simulink model "SteeringWheel"  (R2024b)
settings: configuration reference "STM32H7_Config" (kept outside this file)
libraries: simulink x3
(part 2 of 2)

== stateflow chart SteeringWheel/Overwrite System/BEMSOn ==
  state Map12
    entry:
    BEMSOnOW = 1;
  state Map11
    entry, during:
    BEMSOnOW = 0;
  state Map13
    entry, during:
    BEMSOnOW = -1;
  Map13 -> Map12 [order 2] : after(500,tick)
      | [BSteeringWheelButton3 ==1]
  Map11 -> Map12 [order 1] : after(500,tick)
      | [BSteeringWheelButton4 == 1]
  (default) -> Map13
  Map13 -> Map11 [order 1] : after(500,tick)
      | [BSteeringWheelButton4 ==1]
  Map12 -> Map13 [order 2] : after(500,tick)
      | [BSteeringWheelButton4 ==1]
  Map12 -> Map11 [order 1] : after(500,tick)
      | [BSteeringWheelButton3 == 1]
  Map11 -> Map13 [order 2] : after(500,tick)
      | [BSteeringWheelButton3 ==1]
  data: BSteeringWheelButton3 input double; BSteeringWheelButton4 input double; BEMSOnOW output double

== stateflow chart SteeringWheel/Overwrite System/NThrottleMap ==
  state Map14
    entry:
    NThrottleMapOW = -1;
    PDischargeMaxOW = -1;
    rTorqueSplitOW = -1;
  state Map12
    entry:
    NThrottleMapOW = 1;
    PDischargeMaxOW = 5;
    rTorqueSplitOW = 0.5;
  state Map7
    entry, during:
    NThrottleMapOW = 2;
    PDischargeMaxOW = 78;
    rTorqueSplitOW = 0.8;
  state Map8
    entry, during:
    NThrottleMapOW = 3;
    PDischargeMaxOW = 78;
    rTorqueSplitOW = 0.7;
  state Map9
    entry, during:
    NThrottleMapOW = 4;
    PDischargeMaxOW = 58;
    rTorqueSplitOW = 1;
  state Map10
    entry, during:
    NThrottleMapOW = 5;
    PDischargeMaxOW = 58;
    rTorqueSplitOW = 0.7;
  state Map13
    entry, during:
    NThrottleMapOW = 6;
    PDischargeMaxOW = 38;
    rTorqueSplitOW = 0.7;
  Map8 -> Map9 [order 2] : after(500,tick)
      | [BSteeringWheelButton3 == 1]
  Map10 -> Map13 [order 2] : after(500,tick)
      | [BSteeringWheelButton3 == 1]
  Map9 -> Map10 [order 2] : after(500,tick)
      | [BSteeringWheelButton3 == 1]
  Map7 -> Map8 [order 2] : after(500,tick)
      | [BSteeringWheelButton3 == 1]
  (default) -> Map14
  Map12 -> Map7 [order 2] : after(500,tick)
      | [BSteeringWheelButton3 == 1]
  Map14 -> Map12 [order 1] : after(500,tick)
      | [BSteeringWheelButton3 == 1]
  Map7 -> Map12 [order 1] : after(500,tick)
      | [BSteeringWheelButton4 ==1]
  Map8 -> Map7 [order 1] : after(500,tick)
      | [BSteeringWheelButton4 ==1]
  Map9 -> Map8 [order 1] : after(500,tick)
      | [BSteeringWheelButton4 ==1]
  Map10 -> Map9 [order 1] : after(500,tick)
      | [BSteeringWheelButton4 ==1]
  Map13 -> Map10 [order 1] : after(500,tick)
      | [BSteeringWheelButton4 ==1]
  Map14 -> Map13 [order 2] : after(500,tick)
      | [BSteeringWheelButton4 ==1]
  Map13 -> Map14 [order 2] : after(500,tick)
      | [BSteeringWheelButton3 == 1]
  Map12 -> Map14 [order 1] : after(500,tick)
      | [BSteeringWheelButton4 ==1]
  data: BSteeringWheelButton3 input double; BSteeringWheelButton4 input double; NThrottleMapOW output double; PDischargeMaxOW output double; rTorqueSplitOW output double

== stateflow chart SteeringWheel/NPageSelectorRotary System/Incremental ==
  state Page1
    entry:
    NPage = 1
    old = NPageSelectRotary
  state Page2
    entry:
    NPage = 2
    old = NPageSelectRotary
  state Page3
    entry:
    NPage = 3
    old = NPageSelectRotary
  state Page4
    entry:
    NPage = 4
    old = NPageSelectRotary
  state Page5
    entry:
    NPage = 5
    old = NPageSelectRotary
  state Page6
    entry:
    NPage = 6
    old = NPageSelectRotary
  state Page7
    entry:
    NPage = 7
    old = NPageSelectRotary
  state Page8
    entry:
    NPage = 8
    old = NPageSelectRotary
  state Page9
    entry:
    NPage = 9
    old = NPageSelectRotary
  state Page10
    entry:
    NPage = 10
    old = NPageSelectRotary
  state Page11
    entry:
    NPage = 11
    old = NPageSelectRotary
  Page5 -> Page4 [order 2] : [NPageSelectRotary < old && NPageSelectRotary ~= old]
  Page6 -> Page5 [order 2] : [NPageSelectRotary < old && NPageSelectRotary ~= old]
  Page7 -> Page6 [order 2] : [NPageSelectRotary <= old && NPageSelectRotary ~= old]
  Page9 -> Page8 [order 1] : [NPageSelectRotary < old && NPageSelectRotary ~= old]
  Page10 -> Page9 [order 1] : [NPageSelectRotary < old && NPageSelectRotary ~= old]
  Page11 -> Page10 : [NPageSelectRotary < old && NPageSelectRotary ~= old]
  Page8 -> Page7 [order 1] : [NPageSelectRotary < old && NPageSelectRotary ~= old]
  Page2 -> Page1 [order 1] : [NPageSelectRotary < old && NPageSelectRotary ~= old]
  Page4 -> Page3 [order 2] : [NPageSelectRotary < old && NPageSelectRotary ~= old]
  (default) -> Page1
  Page3 -> Page2 [order 1] : [NPageSelectRotary < old && NPageSelectRotary ~= old]
  Page1 -> Page2 : [NPageSelectRotary > old && NPageSelectRotary ~= old]
  Page2 -> Page3 [order 2] : [NPageSelectRotary > old && NPageSelectRotary ~= old]
  Page3 -> Page4 [order 2] : [NPageSelectRotary > old && NPageSelectRotary ~= old]
  Page4 -> Page5 [order 1] : [NPageSelectRotary > old && NPageSelectRotary ~= old]
  Page5 -> Page6 [order 1] : [NPageSelectRotary > old && NPageSelectRotary ~= old]
  Page6 -> Page7 [order 1] : [NPageSelectRotary > old && NPageSelectRotary ~= old]
  Page7 -> Page8 [order 1] : [NPageSelectRotary > old && NPageSelectRotary ~= old]
  Page8 -> Page9 [order 2] : [NPageSelectRotary > old && NPageSelectRotary ~= old]
  Page9 -> Page10 [order 2] : [NPageSelectRotary > old && NPageSelectRotary ~= old]
  Page10 -> Page11 [order 2] : [NPageSelectRotary > old && NPageSelectRotary ~= old]
  data: old local double; NPage output double; NPageSelectRotary input double

== stateflow chart SteeringWheel/NEventModeRotary System ==
  state Scrut
    entry:
    BTVOnEM = 0
    BTCOnEM = 0
    BDrivetrainCoolingOnEM = 0
    NThrottleMapEM = 1
    PDischargeMaxEM = 5
    rTorqueSplitEM = 0.5
    PRegenMaxEM = 0
    rTVMultiplierEM = 0
    NEventMode = 1
    BEMSOnEM = 0
    BSpinningModeOnEM = 0
    PEngineBrakingEM = 0
    MRegenMax = 0
    rEngineBrakingSplitEM = 1
  state Shakedown
    entry:
    BTVOnEM = 0
    BTCOnEM = 0
    BDrivetrainCoolingOnEM = 1
    NThrottleMapEM = 6
    PDischargeMaxEM = 38
    rTorqueSplitEM = 0.7
    PRegenMaxEM = 20
    rTVMultiplierEM = 0
    NEventMode = 3
    BEMSOnEM = 0
    BSpinningModeOnEM = 0
    PEngineBrakingEM = 6
    MRegenMax = 15
    rEngineBrakingSplitEM = 1
  state Wheelspin
    entry:
    BTVOnEM = 0
    BTCOnEM = 0
    BDrivetrainCoolingOnEM = 0
    NThrottleMapEM = 1
    PDischargeMaxEM = 5
    rTorqueSplitEM = 0.5
    PRegenMaxEM = 0
    rTVMultiplierEM = 0
    NEventMode = 2
    BEMSOnEM = 0
    BSpinningModeOnEM = 1
    PEngineBrakingEM = 0
    MRegenMax = 0
    rEngineBrakingSplitEM = 1
  state Skidpad
    entry:
    BTVOnEM = 1
    BTCOnEM = 1
    BDrivetrainCoolingOnEM = 1
    NThrottleMapEM = 5
    PDischargeMaxEM = 58
    rTorqueSplitEM = 0.7
    PRegenMaxEM = 20
    rTVMultiplierEM = 0.5
    NEventMode = 5
    BEMSOnEM = 0
    BSpinningModeOnEM = 0
    PEngineBrakingEM = 10
    MRegenMax = 60
    rEngineBrakingSplitEM = 1
  state Acceleration
    entry:
    BTVOnEM = 0
    BTCOnEM = 1
    BDrivetrainCoolingOnEM = 1
    NThrottleMapEM = 2
    PDischargeMaxEM = 78
    rTorqueSplitEM = 0.8
    PRegenMaxEM = 0
    rTVMultiplierEM = 0
    NEventMode = 4
    BEMSOnEM = 0
    BSpinningModeOnEM = 0
    PEngineBrakingEM = 0
    MRegenMax = 0
    rEngineBrakingSplitEM = 1
  state Autocross
    entry:
    BTVOnEM = 1
    BTCOnEM = 1
    BDrivetrainCoolingOnEM = 1
    NThrottleMapEM = 3
    PDischargeMaxEM = 78
    rTorqueSplitEM = 0.7
    PRegenMaxEM = 100
    rTVMultiplierEM = 0.5
    NEventMode = 6
    BEMSOnEM = 0
    BSpinningModeOnEM = 0
    PEngineBrakingEM = 14
    MRegenMax = 60
    rEngineBrakingSplitEM = 1
  state Limp
    entry:
    BTVOnEM = 0
    BTCOnEM = 1
    BDrivetrainCoolingOnEM = 1
    NThrottleMapEM = 4
    PDischargeMaxEM = 58
    rTorqueSplitEM = 0.7
    PRegenMaxEM = 0
    rTVMultiplierEM = 0
    NEventMode = 8
    BEMSOnEM = 0
    BSpinningModeOnEM = 0
    PEngineBrakingEM = 0
    MRegenMax = 60
    rEngineBrakingSplitEM = 1
  state Endurance
    entry:
    BTVOnEM = 1
    BTCOnEM = 1
    BDrivetrainCoolingOnEM = 1
    NThrottleMapEM = 3
    PDischargeMaxEM = 78
    rTorqueSplitEM = 0.7
    PRegenMaxEM = 100
    rTVMultiplierEM = 0.5
    NEventMode = 7
    BEMSOnEM = 1
    BSpinningModeOnEM = 0
    PEngineBrakingEM = 14
    MRegenMax = 60
    rEngineBrakingSplitEM = 1
  Scrut -> (junction 31) : after(500, tick)[NEventModeRotary~=1]
  (junction 31) -> Scrut [order 1] : after(500, tick)[NEventModeRotary==1]
  (junction 31) -> Shakedown [order 3] : after(500, tick)[NEventModeRotary==3]
  Wheelspin -> (junction 31) : after(500, tick)[NEventModeRotary~=2]
  (junction 31) -> Wheelspin [order 2] : after(500, tick)[NEventModeRotary==2]
  Shakedown -> (junction 31) : after(500, tick)[NEventModeRotary~=3]
  (junction 31) -> Skidpad [order 4] : after(500, tick)[NEventModeRotary==5]
  Skidpad -> (junction 31) : after(500, tick)[NEventModeRotary~=5]
  Acceleration -> (junction 31) : after(500, tick)[NEventModeRotary~=4]
  (junction 31) -> Acceleration [order 6] : after(500, tick)[NEventModeRotary==4]
  Autocross -> (junction 31) : after(500, tick)[NEventModeRotary~=6]
  (junction 31) -> Limp [order 8] : after(500, tick)[NEventModeRotary==8]
  (junction 31) -> Autocross [order 7] : after(500, tick)[NEventModeRotary==6]
  Limp -> (junction 31) : after(500, tick)[NEventModeRotary~=8]
  Endurance -> (junction 31) : after(500, tick)[NEventModeRotary~=7]
  (junction 31) -> Endurance [order 5] : after(500, tick)[NEventModeRotary==7]
  (default) -> Endurance
  data: BTVOnEM output double; BTCOnEM output double; BDrivetrainCoolingOnEM output double =0; BEMSOnEM output double =0; BSpinningModeOnEM output double; NEventModeRotary input double [0..9]; NThrottleMapEM output double =0; PDischargeMaxEM output double =0; rTorqueSplitEM output double; PRegenMaxEM output double; rTVMultiplierEM output double; PEngineBrakingEM output double = 14; MRegenMax output double =15; rEngineBrakingSplitEM output double =1; NEventMode output double

== stateflow chart SteeringWheel/Overwrite System/BSpinningModeOn ==
  state Map14
    entry:
    BSpinningModeOnOW = 1;
  state Map16
    entry:
    BSpinningModeOnOW = 0;
  state Map15
    entry:
    BSpinningModeOnOW = -1;
  Map15 -> Map14 [order 2] : after(500,tick)
      | [BSteeringWheelButton3 ==1]
  Map14 -> Map16 [order 2] : after(500,tick)
      | [BSteeringWheelButton3 == 1]
  Map15 -> Map16 [order 1] : after(500,tick)
      | [BSteeringWheelButton4 ==1]
  (default) -> Map15
  Map14 -> Map15 [order 1] : after(500,tick)
      | [BSteeringWheelButton4 ==1]
  Map16 -> Map14 [order 2] : after(500,tick)
      | [BSteeringWheelButton3 == 1]
  Map16 -> Map15 [order 1] : after(500,tick)
      | [BSteeringWheelButton3 ==1]
  data: BSteeringWheelButton3 input double; BSteeringWheelButton4 input double; BSpinningModeOnOW output double

== stateflow chart SteeringWheel/Overwrite System/EOffset ==
  state a
    entry, during:
    EOffset = 0;
  state a2
    entry, during:
    EOffset = -3;
  state a3
    entry, during:
    EOffset = -1.5;
  state a6
    entry, during:
    EOffset = 3;
  state a7
    entry, during:
    EOffset = 4.5;
  state a1
    entry, during:
    EOffset = -4.5;
  state a5
    entry, during:
    EOffset = 1.5;
  a -> a1 [order 1] : after(500,tick)
      | [BSteeringWheelButton3 == 1]
  a3 -> a5 [order 2] : after(500,tick)
      | [BSteeringWheelButton3 == 1]
  a6 -> a7 [order 2] : after(500,tick)
      | [BSteeringWheelButton3 == 1]
  a5 -> a6 [order 2] : after(500,tick)
      | [BSteeringWheelButton3 == 1]
  a2 -> a3 [order 2] : after(500,tick)
      | [BSteeringWheelButton3 == 1]
  (default) -> a
  a1 -> a2 [order 1] : after(500,tick)
      | [BSteeringWheelButton3 == 1]
  a -> a7 [order 2] : after(500,tick)
      | [BSteeringWheelButton4 ==1]
  a7 -> a [order 1] : after(500,tick)
      | [BSteeringWheelButton3 == 1]
  a1 -> a [order 2] : after(500,tick)
      | [BSteeringWheelButton4 ==1]
  a2 -> a1 [order 1] : after(500,tick)
      | [BSteeringWheelButton4 ==1]
  a5 -> a3 [order 1] : after(500,tick)
      | [BSteeringWheelButton4 ==1]
  a6 -> a5 [order 1] : after(500,tick)
      | [BSteeringWheelButton4 ==1]
  a3 -> a2 [order 1] : after(500,tick)
      | [BSteeringWheelButton4 ==1]
  a7 -> a6 [order 2] : after(500,tick)
      | [BSteeringWheelButton4 ==1]
  data: BSteeringWheelButton3 input double; BSteeringWheelButton4 input double; EOffset output double
